simulink model "counter1"  (R2019a)
settings: Solver=FixedStepDiscrete  StartTime=0.0  StopTime=10.0  FixedStep=0.2  RelTol=1e-3
settings Model: Creator=Sagar  LastModifiedBy=Sagar

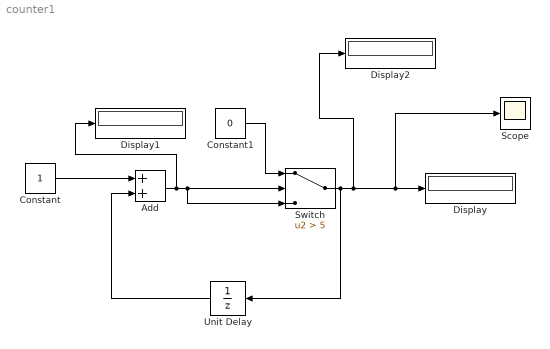
== system counter1 ==
  Add : Sum
  Constant : Constant
  Constant1 : Constant  Value=0
  Display : Display
  Display1 : Display
  Display2 : Display
  Scope : Scope
  Switch : Switch  Criteria=u2 > Threshold  Threshold=5
  Unit Delay : UnitDelay  InitialCondition=-1  SampleTime=-1  HasFrameUpgradeWarning=on
  wires:
  Constant/1 -> Add/1
  Add/1 -> Display1/1, Switch/3, Switch/2
  Constant1/1 -> Switch/1
  Switch/1 -> Unit Delay/1, Display2/1, Scope/1, Display/1
  Unit Delay/1 -> Add/2
